simulink model "unicycle_singularity_check"  (R2023b)
settings: Solver=ode45  StartTime=0.0  StopTime=40  MaxStep=0.01  RelTol=1e-3
values from neighbouring files (symbols this model uses):
  initial_condition = [12 0 pi/2]    [initialize.m]
  parking_spot = [14 0 -pi/2]    [initialize.m]
  use_posture_regulator = 1    [initialize.m]
libraries: dspsigops x1
settings Model: Creator=utente  LastModifiedBy=ricca
settings DataIOCC: ReturnWorkspaceOutputs=off

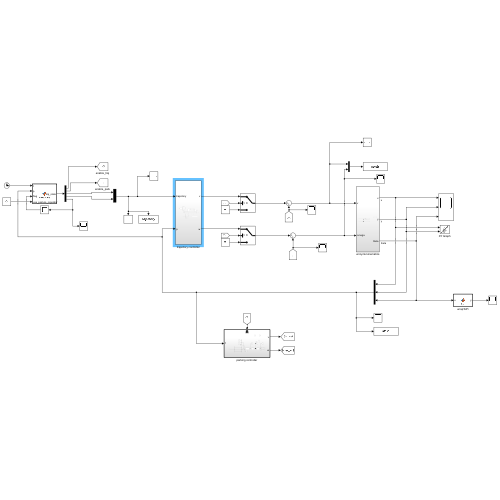
[thumbnail: Simulink's stored preview of the top-level diagram]
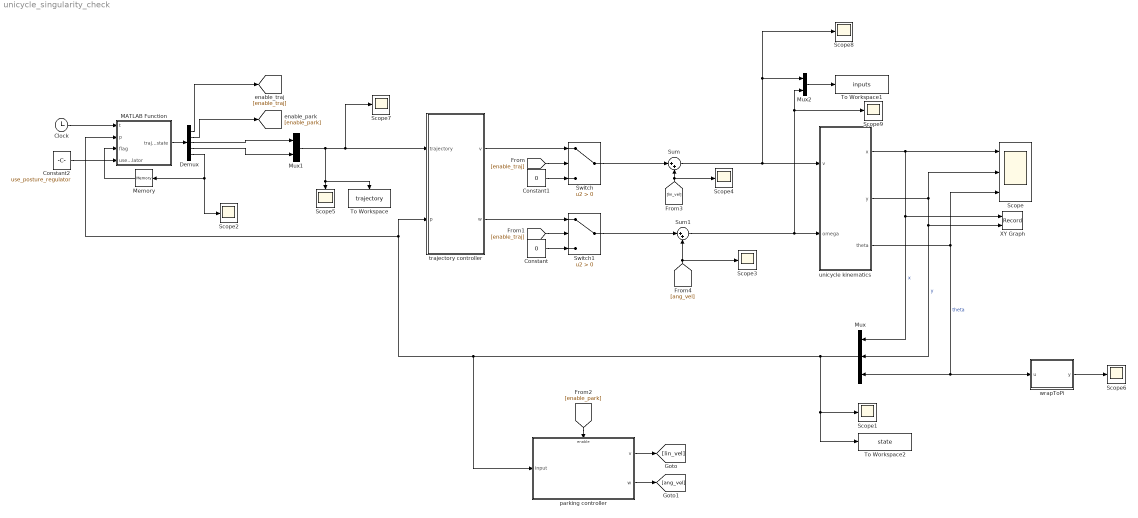
== system unicycle_singularity_check ==
  Clock : Clock
  Constant : Constant  Value=0
  Constant1 : Constant  Value=0
  Constant2 : Constant  Value=use_posture_regulator
  Demux : Demux  Outputs=5
  MATLAB Function : MATLAB Function  TreatAsAtomicUnit=on
  Memory : Memory  InitialCondition=1
  Mux : Mux  Inputs=3
  Mux1 : Mux  Inputs=2
  Mux2 : Mux  Inputs=2
  Scope : Scope  NumInputPorts=3
  Scope{1..9} (9 alike) : Scope
  Sum : Sum  Inputs=|++
  Sum1 : Sum  Inputs=|++
  Switch : Switch  Criteria=u2 > Threshold  SaturateOnIntegerOverflow=off  InputSameDT=off
  Switch1 : Switch  Criteria=u2 > Threshold  SaturateOnIntegerOverflow=off  InputSameDT=off
  To Workspace : ToWorkspace  VariableName=trajectory  SaveFormat=Structure With Time  SampleTime=-1
  To Workspace1 : ToWorkspace  VariableName=inputs  SaveFormat=Structure With Time  SampleTime=-1
  To Workspace2 : ToWorkspace  VariableName=state  SaveFormat=Structure With Time  SampleTime=-1
  XY Graph : Record  FileSettingsInternal="{\"entries\":[{\"content\":{\"excelSettings\":{\"content\":{},\"type\":\"Streamout.ExcelSettings\"}},\"type\":\"Streamout.FileSettingStorage\",\"uuid\":\"\"}],\"packageUris\":[\"http:\\/\\/schema.mathworks.com\\/mf0\\/streamout_blocks\\/R2020a\"],\"version\":\"1.0\"}"  Layout=[1 1]  SignalsInternal="{\"entries\":[{\"content\":{\"signals\":[{\"content\":{\"blockPath\":[],\"dimensions\":[1,1],\"domain\":\"\",\"lineColor\":\"#a2142f\",\"plots\":[ 1 ],\"port\":1,\"sid\":[\"\"],\"signalID\":1,\"signalName\":\"x\"},\"type\":\"RecordBlkView.Signal\",\"uuid\":\"\"},{\"content\":{\"blockPath\":[],\"dimensions\":[1,1],\"domain\":\"\",\"lineColor\":\"#139fff\",\"plots\":[ 1 ],\"port\":2,\"sid\":[\"\"],\"signalID\":2,\"signalName\":\"y\"},\"type\":\"RecordBlkView.Signal\",\"uuid\":\"\"}]},\"type\":\"RecordBlkView.InputSignals\",\"uuid\":\"\"}],\"packageUris\":[\"http:\\/\\/schema.mathworks.com\\/mf0\\/streamout_blocks\\/R2020a\"],\"version\":\"1.0\"}"  VisualizationBindings="{\"xyplotplugin\":{\"info\":[{\"series\":[{\"bindingParametersList\":[{\"parameter\":\"X-Axis\",\"signalID\":1,\"signalName\":\"x\"},{\"parameter\":\"Y-Axis\",\"signalID\":2,\"signalName\":\"y\"}],\"seriesID\":0}],\"subplotID\":1}]}}"  CompatibilityTag=XY
  parking controller : Subsystem
  trajectory controller : Subsystem
  unicycle kinematics : Subsystem
  wrapToPi : MATLAB Function  TreatAsAtomicUnit=on
  wires:
  unicycle kinematics/1(x) -> Mux/1, XY Graph/1, Scope/1  "x"
  unicycle kinematics/2(y) -> Mux/2, XY Graph/2, Scope/2  "y"
  unicycle kinematics/3(theta) -> Mux/3, wrapToPi/1(u), Scope/3  "theta"
  Sum1/1 -> Scope9/1, Mux2/2, unicycle kinematics/2(omega)
  Sum/1 -> unicycle kinematics/1(v), Scope8/1, Mux2/1
  trajectory controller/1(v) -> Switch/1
  trajectory controller/2(w) -> Switch1/1
  Mux/1 -> Scope1/1, To Workspace2/1, parking controller/1(Input), MATLAB Function/2(p), trajectory controller/2(p)
  MATLAB Function/1(traj_state) -> Demux/1
  Demux/3 -> Mux1/1
  Demux/4 -> Mux1/2
  Mux1/1 -> Scope7/1, trajectory controller/1(trajectory), To Workspace/1, Scope5/1
  Clock/1 -> MATLAB Function/1(t)
  Memory/1 -> MATLAB Function/3(flag)
  Demux/5 -> Scope2/1, Memory/1
  Switch/1 -> Sum/1
  Switch1/1 -> Sum1/1
  Constant/1 -> Switch1/3
  Constant1/1 -> Switch/3
  Demux/1 -> [enable_traj]
  [enable_traj] -> Switch/2
  [enable_traj] -> Switch1/2
  Demux/2 -> [enable_park]
  [enable_park] -> parking controller/Enable
  parking controller/1(v) -> [lin_vel]
  parking controller/2(w) -> [ang_vel]
  [lin_vel] -> Scope4/1, Sum/2
  [ang_vel] -> Sum1/2, Scope3/1
  wrapToPi/1(y) -> Scope6/1
  Mux2/1 -> To Workspace1/1
  Constant2/1 -> MATLAB Function/4(use_posture_regulator)

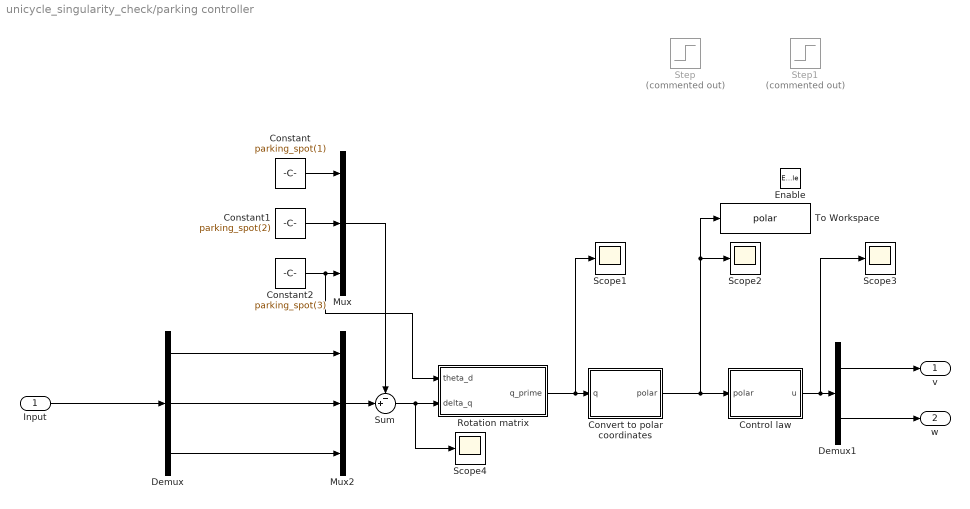
== system unicycle_singularity_check/parking controller ==
  Input : Inport
  Enable : EnablePort  StatesWhenEnabling=reset
  Constant : Constant  Value=parking_spot(1)
  Constant1 : Constant  Value=parking_spot(2)
  Constant2 : Constant  Value=parking_spot(3)
  Control law : MATLAB Function  TreatAsAtomicUnit=on
  Convert to polar coordinates : MATLAB Function  TreatAsAtomicUnit=on
  Demux : Demux  Outputs=3
  Demux1 : Demux  Outputs=2
  Mux : Mux  Inputs=3
  Mux2 : Mux  Inputs=3
  Rotation matrix : MATLAB Function  TreatAsAtomicUnit=on
  Scope{1..4} (4 alike) : Scope
  Step : Step  Commented=on  SampleTime=0
  Step1 : Step  Commented=on  After=0  SampleTime=0
  Sum : Sum  Inputs=-+|
  To Workspace : ToWorkspace  VariableName=polar  SaveFormat=Structure With Time  SampleTime=-1
  v : Outport
  w : Outport  Port=2
  wires:
  Rotation matrix/1(q_prime) -> Scope1/1, Convert to polar coordinates/1(q)
  Demux1/2 -> w/1
  Constant2/1 -> Rotation matrix/1(theta_d), Mux/3
  Constant1/1 -> Mux/2
  Mux2/1 -> Sum/2
  Mux/1 -> Sum/1
  Sum/1 -> Scope4/1, Rotation matrix/2(delta_q)
  Demux1/1 -> v/1
  Convert to polar coordinates/1(polar) -> Control law/1(polar), To Workspace/1, Scope2/1
  Constant/1 -> Mux/1
  Control law/1(u) -> Scope3/1, Demux1/1
  Input/1 -> Demux/1
  Demux/2 -> Mux2/2
  Demux/1 -> Mux2/1
  Demux/3 -> Mux2/3

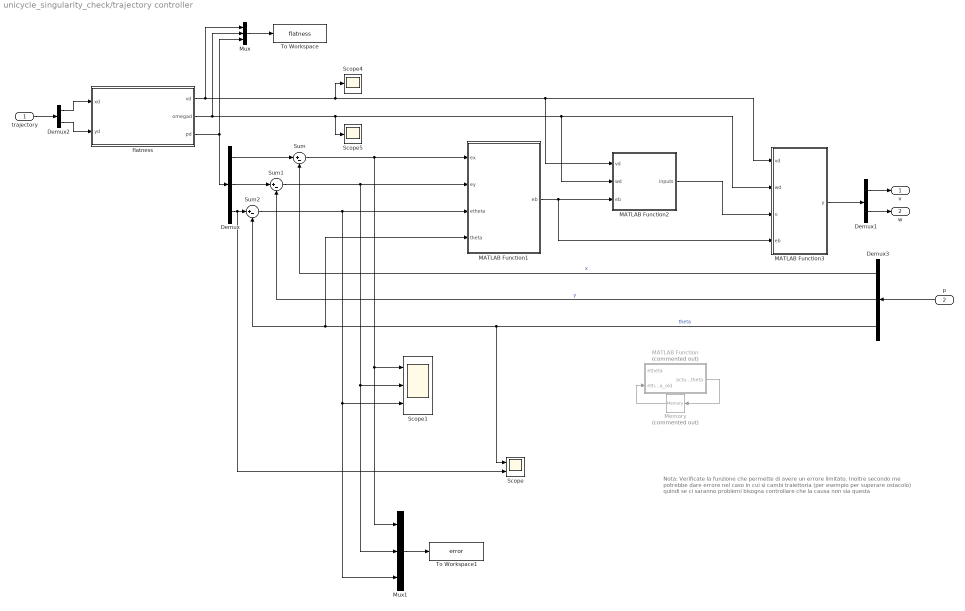
== system unicycle_singularity_check/trajectory controller ==
  note: Nota: Verificate la funzione che permette di avere un errore limitato. Inoltre secondo me potrebbe dare errore nel caso in cui si cambi traiettoria (per esempio per superare ostacolo) quindi se ci saranno problemi bisogna controllare che la causa non sia questa
  trajectory : Inport
  p : Inport  Port=2
  Demux : Demux  Outputs=3
  Demux1 : Demux  Outputs=2
  Demux2 : Demux  Outputs=2
  Demux3 : Demux  Outputs=3
  MATLAB Function : MATLAB Function  Commented=on  TreatAsAtomicUnit=on
  MATLAB Function1 : MATLAB Function  TreatAsAtomicUnit=on
  MATLAB Function2 : MATLAB Function  TreatAsAtomicUnit=on
  MATLAB Function3 : MATLAB Function  TreatAsAtomicUnit=on
  Memory : Memory  Commented=on  InitialCondition=1
  Mux : Mux  Inputs=3
  Mux1 : Mux  Inputs=3
  Scope : Scope  NumInputPorts=2
  Scope1 : Scope  NumInputPorts=3
  Scope4 : Scope
  Scope5 : Scope
  Sum : Sum  Inputs=|+-
  Sum1 : Sum  Inputs=|+-
  Sum2 : Sum  Inputs=|+-
  To Workspace : ToWorkspace  VariableName=flatness  SaveFormat=Structure With Time  SampleTime=-1
  To Workspace1 : ToWorkspace  VariableName=error  SaveFormat=Structure With Time  SampleTime=-1
  flatness : Subsystem
  v : Outport
  w : Outport  Port=2
  wires:
  Demux/1 -> Sum/1
  Demux/3 -> Scope/2, Sum2/1
  MATLAB Function2/1(inputs) -> MATLAB Function3/3(u)
  Demux3/3 -> Scope/1, MATLAB Function1/4(theta), Sum2/2  "theta"
  Sum1/1 -> Mux1/2, Scope1/2, MATLAB Function1/2(ey)
  Sum/1 -> Mux1/1, Scope1/1, MATLAB Function1/1(ex)
  Demux1/1 -> v/1
  flatness/1(vd) -> MATLAB Function2/1(vd), MATLAB Function3/1(vd), Scope4/1, Mux/1
  MATLAB Function3/1(y) -> Demux1/1
  Sum2/1 -> Mux1/3, Scope1/3, MATLAB Function1/3(etheta)
  flatness/2(omegad) -> Scope5/1, MATLAB Function2/2(wd), MATLAB Function3/2(wd), Mux/2
  flatness/3(pd) -> Mux/3, Demux/1
  Demux3/1 -> Sum/2  "x"
  MATLAB Function1/1(eb) -> MATLAB Function2/3(eb), MATLAB Function3/4(eb)
  Demux1/2 -> w/1
  Demux/2 -> Sum1/1
  Demux2/2 -> flatness/2(yd)
  Demux2/1 -> flatness/1(xd)
  Demux3/2 -> Sum1/2  "y"
  trajectory/1 -> Demux2/1
  p/1 -> Demux3/1
  MATLAB Function/1(actual_etheta) -> Memory/1
  Memory/1 -> MATLAB Function/2(etheta_old)
  Mux/1 -> To Workspace/1
  Mux1/1 -> To Workspace1/1

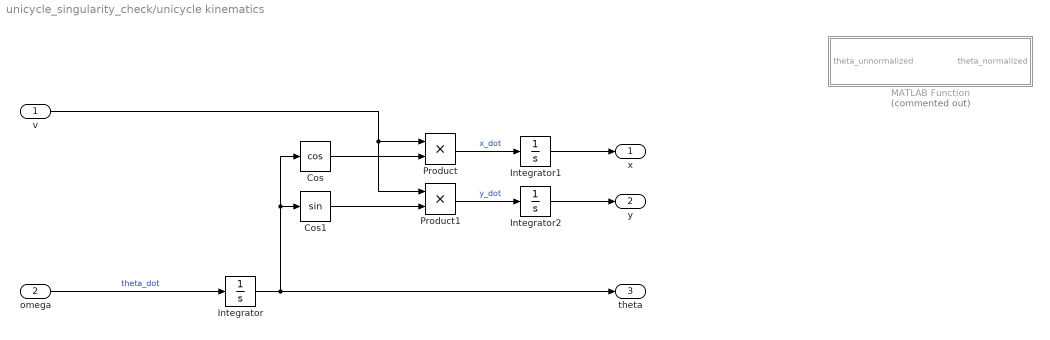
== system unicycle_singularity_check/unicycle kinematics ==
  v : Inport
  omega : Inport  Port=2
  Cos : Trigonometry  Operator=cos
  Cos1 : Trigonometry
  Integrator : Integrator  InitialCondition=initial_condition(3)  ZeroCross=off
  Integrator1 : Integrator  InitialCondition=initial_condition(1)
  Integrator2 : Integrator  InitialCondition=initial_condition(2)
  MATLAB Function : MATLAB Function  Commented=on  TreatAsAtomicUnit=on
  Product : Product
  Product1 : Product
  x : Outport
  y : Outport  Port=2
  theta : Outport  Port=3
  wires:
  Integrator/1 -> theta/1, Cos/1, Cos1/1
  Integrator2/1 -> y/1
  Cos1/1 -> Product1/2
  Product/1 -> Integrator1/1  "x_dot"
  v/1 -> Product/1, Product1/1
  Product1/1 -> Integrator2/1  "y_dot"
  omega/1 -> Integrator/1  "theta_dot"
  Integrator1/1 -> x/1
  Cos/1 -> Product/2

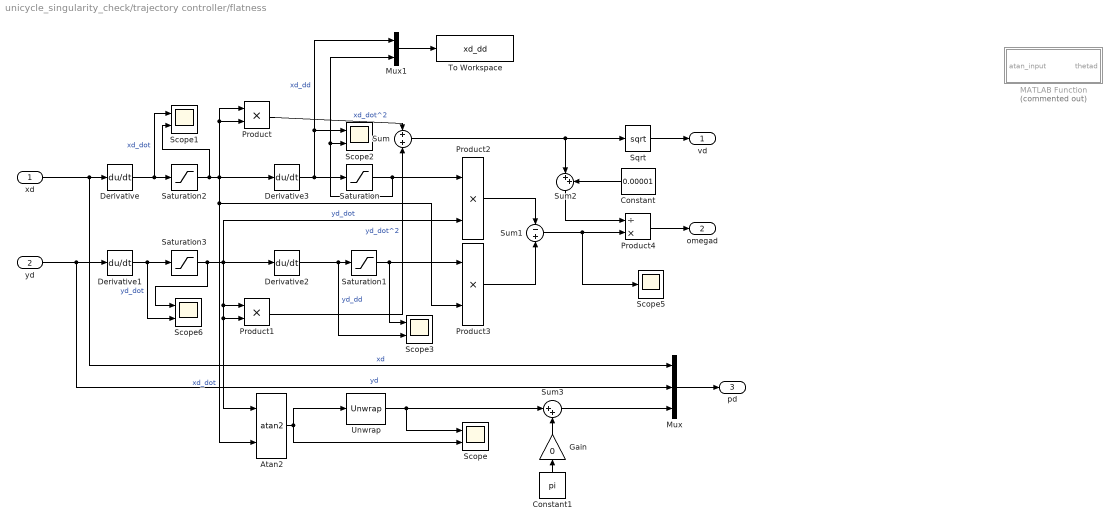
== system unicycle_singularity_check/trajectory controller/flatness ==
  xd : Inport
  yd : Inport  Port=2
  Atan2 : Trigonometry  Operator=atan2
  Constant : Constant  Value=0.00001
  Constant1 : Constant  Value=pi
  Derivative{,1..3} (4 alike) : Derivative
  Gain : Gain  Gain=0
  MATLAB Function : MATLAB Function  Commented=on  TreatAsAtomicUnit=on
  Mux : Mux  Inputs=3
  Mux1 : Mux  Inputs=2
  Product{,1..3} (4 alike) : Product
  Product4 : Product  Inputs=/*
  Saturation{,1..3} (4 alike) : Saturate  UpperLimit=2.5  LowerLimit=-2.5  ZeroCross=off
  Scope{,1..3,6} (5 alike) : Scope  NumInputPorts=2
  Scope5 : Scope
  Sqrt : Sqrt
  Sum : Sum  Inputs=+|+
  Sum1 : Sum  Inputs=-|+
  Sum2 : Sum  Inputs=|++
  Sum3 : Sum  Inputs=|++
  To Workspace : ToWorkspace  VariableName=xd_dd  SaveFormat=Structure With Time  SampleTime=-1
  Unwrap : dspsigops/Unwrap  tol=pi  InputProcessing=Columns as channels (frame based)  running=off
  vd : Outport
  omegad : Outport  Port=2
  pd : Outport  Port=3
  wires:
  xd/1 -> Derivative/1, Mux/1  "xd"
  yd/1 -> Derivative1/1, Mux/2  "yd"
  Derivative/1 -> Scope1/1, Saturation2/1  "xd_dot"
  Derivative1/1 -> Scope6/2, Saturation3/1  "yd_dot"
  Product/1 -> Sum/1  "xd_dot^2"
  Product1/1 -> Sum/2  "yd_dot^2"
  Sum/1 -> Sum2/1, Sqrt/1
  Sqrt/1 -> vd/1
  Product2/1 -> Sum1/1
  Product3/1 -> Sum1/2
  Sum1/1 -> Scope5/1, Product4/2
  Product4/1 -> omegad/1
  Sum2/1 -> Product4/1
  Constant/1 -> Sum2/2
  Atan2/1 -> Unwrap/1, Scope/2
  Constant1/1 -> Gain/1
  Gain/1 -> Sum3/2
  Sum3/1 -> Mux/3
  Mux/1 -> pd/1
  Unwrap/1 -> Scope/1, Sum3/1
  Derivative3/1 -> Mux1/1, Scope2/1, Saturation/1  "xd_dd"
  Saturation/1 -> Scope2/2, Mux1/2, Product2/1
  Derivative2/1 -> Scope3/2, Saturation1/1  "yd_dd"
  Saturation1/1 -> Scope3/1, Product3/1
  Saturation2/1 -> Scope1/2, Product3/2, Atan2/2, Derivative3/1, Product/2, Product/1  "xd_dot"
  Saturation3/1 -> Scope6/1, Atan2/1, Product1/2, Product1/1, Product2/2, Derivative2/1  "yd_dot"
  Mux1/1 -> To Workspace/1

== matlab function unicycle_singularity_check/trajectory controller/flatness/MATLAB Function ==
  data: atan_input input; thetad output
function thetad = convert_angle(atan_input)
    if(atan_input < 0)
        thetad = atan_input + 2*pi;
    else
        thetad = atan_input;
    end

== matlab function unicycle_singularity_check/MATLAB Function ==
  data: t input; traj_state output; p input; flag input; use_posture_regulator input
function traj_state= trajectory(t,p,flag, use_posture_regulator)
r1 = 10; % trajectory radius
r2 = 1;  % obstacle avoidance trajectory radius
r3 = 2;  % parking maneuver radius
omega = 0.3;
traj_state = zeros(5,1);

enable_traj = 0;
enable_park = 0;
x = 0;
y = 0;

% First quarter of circle
if(flag == 1)
    enable_traj = 1;
    enable_park = 0;
    x = r1*cos(omega*t);
    y = r1*sin(omega*t);
end

if(abs(p(1))<1 && abs(p(2) - r1)<1 && flag==1)
    enable_traj = 1;
    enable_park = 0;
    flag = 2;
end

% Obstacle avoidance
if(flag==2)
    enable_traj = 1;
    enable_park = 0;
    x = r2*cos(omega*(t-5));%5
    y = r1 + r2*sin(omega*(t-5));%pi/2
end
if(abs(p(1) + r2)<0.1 && abs(p(2) - r1)<0.1 && flag==2)
    enable_traj = 0;
    enable_park = 1;
    flag = 3;
end

% Last 3/4 of a circle
if(flag==3)
    enable_traj = 1;
    enable_park = 0;
    x = r1*cos(omega*(t - 15) + 1.67);%15
    y = r1*sin(omega*(t - 15) + 1.67);%4.6
end

% Park
if(t>4 && abs(p(1)-r1)<0.25 && abs(p(2))<0.25 && flag==3)
    if(use_posture_regulator==1)
        flag = 4;
        enable_traj = 0;
        enable_park = 1;
    else
        flag = 5;
    end
end

% if(t>2 && abs(p(1)-r)<0.01 && abs(p(2))<0.01 && flag==1)
%     enable_traj = 0;
%     enable_park = 1;
%     flag = 2;
% % end
% if(t>2 && abs(p(1)-r)<0.1 && abs(p(2))<0.1 && flag==1)%prova
%     enable_traj = 1;
%     enable_park = 0;
%     flag = 2;
% end
% if(flag==2)
%     enable_traj = 1;
%     enable_park = 0;
%     x = r + t-2*pi;
%     y = 0;
% end
if(flag==4)
    enable_traj = 0;
    enable_park = 1;
end

if(flag == 5)
    enable_traj = 1;
    enable_park = 0;
    x = 12-r3*cos(omega*(t-9.1));
    y = r3*sin(omega*(t-9.1));
end

flag_out= flag;

traj_state = [enable_traj;enable_park;x;y;flag_out];

== matlab function unicycle_singularity_check/unicycle kinematics/MATLAB Function ==
  data: theta_unnormalized input; theta_normalized output
function theta_normalized = normalize_theta(theta_unnormalized)

    theta_normalized = mod(theta_unnormalized, 2*pi);

== matlab function unicycle_singularity_check/trajectory controller/MATLAB Function1 ==
  data: ex input; eb output; ey input; etheta input; theta input
function eb = fcn(ex,ey,etheta,theta)
    M = [cos(theta),sin(theta),0; -sin(theta),cos(theta),0; 0,0,1];
    eb = M*[ex;ey;etheta];

== matlab function unicycle_singularity_check/trajectory controller/MATLAB Function2 ==
  data: inputs output; vd input; wd input; eb input
function inputs = fcn(vd,wd,eb)
d = 0.4;%csi
a = 8;
k1 = 2*d*a;
if abs(vd) < 1e-4
    if vd >= 0
        vd = 1e-4;
    else
        vd =-1e-4;
    end
end
k2 = (a^2- wd^2)/vd;
k3 = k1;
k = [-k1,0,0;0,-k2,-k3];
inputs = k*eb;

== matlab function unicycle_singularity_check/trajectory controller/MATLAB Function3 ==
  data: vd input; y output; wd input; u input; eb input
function y= fcn(vd,wd,u,eb)
y=zeros(1,2);
y(1) = vd*cos(eb(3)) - u(1);
y(2) = wd - u(2);

== matlab function unicycle_singularity_check/trajectory controller/MATLAB Function ==
  data: etheta input; actual_etheta output; etheta_old input
function actual_etheta = fcn(etheta,etheta_old)

if(etheta-etheta_old > 4)
    actual_etheta = etheta - 2*pi; 
elseif(etheta-etheta_old < -4)
    actual_etheta = etheta + 2*pi;
else
    actual_etheta = etheta;
end

== matlab function unicycle_singularity_check/parking controller/Control law ==
  data: polar input; u output
function u = fcn(polar)
u = zeros(2,1);

rho = polar(1);
gamma = polar(2);
delta = polar(3);

k1 = 3;
k2 = 3;
k3 = 3;

v = k1*rho*cos(gamma);

if (abs(gamma) > 0.0001 && rho > 0.0001)
    w = k2*gamma+(k1*sin(gamma)*cos(gamma)/gamma*(gamma+k3*delta));
else
    w = 0;
    v = 0;
end
u = [v;w];

== matlab function unicycle_singularity_check/parking controller/Convert to polar coordinates ==
  data: q input; polar output
function polar = fcn(q)
polar = zeros(3,1);

rho = sqrt(q(1)^2+q(2)^2);
gamma = atan2(q(2),q(1)) + pi - q(3);
delta = gamma + q(3);

polar = [rho; wrapToPi(gamma); wrapToPi(delta)];

% I need to wrap between [-pi, +pi] so that when we are stabilizing
% around 0 we do not continuously switch between 0 and 2pi.
% Here I must not unwrap the angles because the angles are used as 
% multipliers in the computation of w, so they need to be expressed in
% normalized radians.

== matlab function unicycle_singularity_check/parking controller/Rotation matrix ==
  data: theta_d input; delta_q input; q_prime output
% I need to express polar coordinates with respect to a rotated frame.
% The rotated frame is obtained by rotating about the z axis of the 
% original one by theta_d radians. 
% So, to express delta_q in that rotated frame I need to change the basis 
% from the original one to the rotated one, and so I multiply delta_q by 
% the inverted (= transposed) rotation matrix.
function q_prime = fcn(theta_d,delta_q)
c = cos(theta_d);
s = sin(theta_d);

% Rotation matrix
R = [c  s   0;
     -s c   0;
     0  0   1];

q_prime = R*delta_q;

== matlab function unicycle_singularity_check/wrapToPi ==
  data: u input; y output
% Just to display the unicycle angle in a more intuitive way
function y = fcn(u)

y = wrapToPi(u);
